simulink model "complex_convert_blk"  (R2019a)
settings: Solver=VariableStepAuto  StartTime=0.0  StopTime=10.0  RelTol=1e-3
libraries: xbsIndex_r4 x2
settings Model: Creator=mybur  LastModifiedBy=mybur

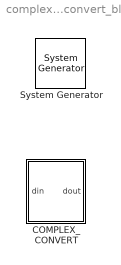
== system complex_convert_blk ==
  " System Generator" : xbsIndex_r4/ System Generator  Tag=genX  xilinxfamily=kintex7  part=xc7k325t  speed=-3  package=fbg676  synthesis_tool=Vivado  clock_wrapper=Clock Enables  directory=./netlist  proj_type=Vivado  Synth_file=Vivado Synthesis Defaults  Impl_file=Vivado Implementation Defaults  testbench=off  simulink_period=1  sysclk_period=10  dcm_input_clock_period=10  incr_netlist=off  trim_vbits=Everywhere in SubSystem  dbl_ovrd=According to Block Masks  core_generation=According to Block Masks  run_coregen=off  deprecated_control=off  eval_field=0  block_type=sysgen
  COMPLEX_CONVERT : Subsystem  mask(complex_convert){n_bits_in=10, bin_pt_in=5, n_bits_out=8, bin_pt_out=4, quantization=Round  (unbiased: +/- Inf), overflow=Wrap, csp_latency=2}
      mask prompts: n_bits_in "Bit Width In"; bin_pt_in "Binary Point In"; n_bits_out "Bit Width Out"; bin_pt_out "Binary Point Out"; csp_latency "Latency"
      mask help: Convert real and imaginary components of a complex input to the specified bit width and precision.
      mask init:
      | Simulink.Block.eval([gcb, '/complex_convert']);
      mask TypeOptions quantization: Truncate | Round  (unbiased: +/- Inf) | Round  (unbiased: Even Values)
      mask TypeOptions overflow: Wrap | Saturate

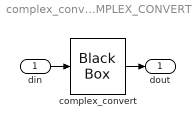
== system complex_convert_blk/COMPLEX_CONVERT ==
  din : Inport
  complex_convert : xbsIndex_r4/Black Box  init_code=complex_convert_config  sim_method=ISE Simulator  verbose=off  block_type=blackbox2
  dout : Outport
  wires:
  din/1 -> complex_convert/1
  complex_convert/1 -> dout/1
